simulink model "buck_mppt"  (R2020a)
settings: Solver=FixedStepAuto  StartTime=0.0  StopTime=sim_duration  FixedStep=sample_time  RelTol=1e-3
values from neighbouring files (symbols this model uses):
  Cin = 300e-6    (= 0.0003)    [main.m]
  Cout = delta_IL / (8 * fsw * delta_Vout)    (= 0.000115)    [main.m]
  delay = 0e-6    (= 0)    [main.m]
  duty_init = 0.4    [main.m]
  fsw = 1e4    (= 10000)    [main.m]
  Irradiance = 1000    [main.m]
  L = Vout * (Vin - Vout) / (delta_IL * fsw * Vin)    (= 0.000839920948617)    [main.m]
  r_small = 1e-3    (= 0.001)    [main.m]
  sample_time = 1e-6    (= 1e-06)    [main.m]
  Temperature = 25    [main.m]
  Voc = 21.9    [main.m]
  Vout = 4    [main.m]
libraries: powerlib x10, powerlib_meascontrol x3, simulink x2, re_lib x1, eePwmGenerator x1
settings Model: Creator=HP  LastModifiedBy=HP

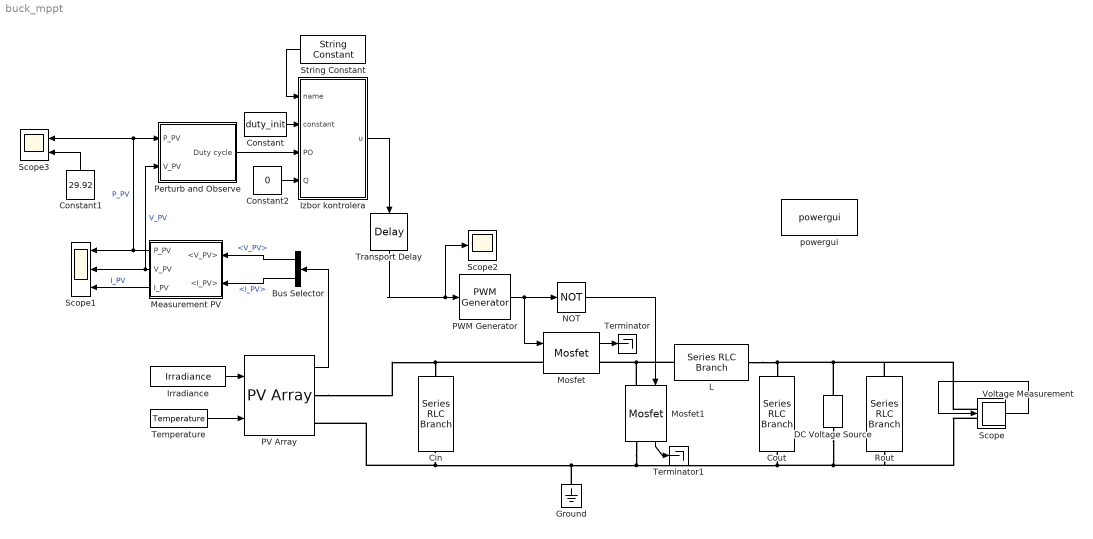
== system buck_mppt ==
  Bus Selector : BusSelector  OutputSignals=V_PV,I_PV
  Cin : powerlib/Elements/Series RLC Branch  LConnTagsString=__new0  RConnTagsString=__new0  BranchType=RC  Resistance=r_small  Inductance=L  SetiL0=off  InitialCurrent=0  Capacitance=Cin  Setx0=on  InitialVoltage=15  Measurements=None
  Constant : Constant  Value=duty_init
  Constant1 : Constant  Value=29.92
  Constant2 : Constant  Value=0
  Cout : powerlib/Elements/Series RLC Branch  LConnTagsString=__new0  RConnTagsString=__new0  BranchType=RC  Resistance=r_small  Inductance=L  SetiL0=off  InitialCurrent=0  Capacitance=Cout  Setx0=off  InitialVoltage=0  Measurements=None
  DC Voltage Source : powerlib/Electrical Sources/DC Voltage Source  Amplitude=Vout  Measurements=None
  Ground : powerlib/Elements/Ground  LConnTagsString=a
  Irradiance : Constant  Value=Irradiance
  Izbor kontrolera : Subsystem
  L : powerlib/Elements/Series RLC Branch  LConnTagsString=__new0  RConnTagsString=__new0  BranchType=RL  Resistance=r_small  Inductance=L  SetiL0=off  InitialCurrent=0  Capacitance=1e-6  Setx0=off  InitialVoltage=0  Measurements=None
  Measurement PV : Subsystem
  Mosfet : powerlib/Power Electronics/Mosfet  Ron=0.1  Lon=0  Rd=0.01  Vfd=0  IC=0  Rs=1e5  Cs=inf  Measurements=on
  Mosfet1 : powerlib/Power Electronics/Mosfet  Ron=0.1  Lon=0  Rd=0.01  Vfd=0  IC=0  Rs=1e5  Cs=inf  Measurements=on
  NOT : Logic  Operator=NOT  IconShape=distinctive  AllPortsSameDT=off  OutDataTypeStr=boolean
  PV Array : re_lib/Solar/PV Array  Npar=1  Nser=1  PlotType=array @ 1000 W/m2 & specified temperatures  S_vec="[ 1000  500  100 ]"  Temp_C_vec="[ 45 25  ]"  ModuleName=User-defined  PlotWhenSelected=off  Pm=29.92  Ncell=36  Voc=21.9  Isc=1.84  Vm=17.6  Im=1.7  beta_Voc_pc=-0.36099  alpha_Isc_pc=0.102  beta_Voc=-0.079057  alpha_Isc=0.0018768  IL=1.8445  I0=6.8285e-11  nI=0.98705  Rsh=385.9657  Rs=0.95187  RobustModel=off  RobustCellTemperature=Temperature  BAL=on  Tc=1e-6  Tfilter=5e-5
  PWM Generator : eePwmGenerator/PWM Generator  CarrCount=Up  Tper=1/fsw  Ts=sample_time
  Perturb and Observe : Subsystem
  Rout : powerlib/Elements/Series RLC Branch  LConnTagsString=__new0  RConnTagsString=__new0  BranchType=R  Resistance=1  Inductance=L  SetiL0=off  InitialCurrent=0  Capacitance=Cout  Setx0=off  InitialVoltage=0  Measurements=None
  Scope : Scope
  Scope1 : Scope  NumInputPorts=3
  Scope2 : Scope
  Scope3 : Scope  NumInputPorts=2
  String Constant : StringConstant  String=mppt_algo_name
  Temperature : Constant  Value=Temperature
  Terminator : Terminator
  Terminator1 : Terminator
  Transport Delay : TransportDelay  DelayTime=delay
  Voltage Measurement : powerlib/Measurements/Voltage Measurement  PhasorSimulation=off  OutputType=Complex  PSBequivalent=0
  powergui : powerlib/powergui  Priority=1  SimulationMode=Discrete  SampleTime=sample_time  frequency=60  Iterations=50  frequencyindice=0  Pbase=100e6  ErrMax=1e-4  UnitsV=kV  UnitsW=MW  buscounter=0  FunctionMessages=off  echomessages=off  EnableUseOfTLC=off  CurrentSourceSwitches=off  DisableSnubberDevices=off  DisableRonSwitches=off  DisableVfSwitches=off  DisplayEquations=off  AutomaticDiscreteSolvers=off  SolverType=Tustin/Backward Euler (TBE)  Interpol=off  ExternalGateDelay=off  methode=off  Ts=100  x0status=blocks  SPID=on  SwTol=0  HookPort=off  NonlinearTolerance=1e-4  nMaxIteration=100  ContinueOnMaxIteration=off  RestoreLinks=warning  ResistiveCurrentMeasurement=off  Frange=[0:2:500]  Ylog=off  Xlog=on  ShowGrid=off  save=off  variable=ZData  structure=0  ZoomFFT=off  StartTime=0.0  cycles=1  DisplayStyle=1  fundamental=60  FreqAxis=off  MaxFrequency=1000  frequencyindicesteady=1  RmsSteady=1  display=off
  wires:
  PWM Generator/1 -> NOT/1, Mosfet/1
  NOT/1 -> Mosfet1/1
  Mosfet/1 -> Terminator/1
  Mosfet1/1 -> Terminator1/1
  Voltage Measurement/1 -> Scope/1
  Irradiance/1 -> PV Array/1
  Temperature/1 -> PV Array/2
  PV Array/1 -> Bus Selector/1
  Bus Selector/1 -> Measurement PV/1(<V_PV>)  "<V_PV>"
  Bus Selector/2 -> Measurement PV/2(<I_PV>)  "<I_PV>"
  Measurement PV/1(P_PV) -> Perturb and Observe/1(P_PV), Scope3/1, Scope1/1  "P_PV"
  Measurement PV/2(V_PV) -> Perturb and Observe/2(V_PV), Scope1/2  "V_PV"
  Measurement PV/3(I_PV) -> Scope1/3  "I_PV"
  Constant1/1 -> Scope3/2
  String Constant/1 -> Izbor kontrolera/1(name)
  Constant/1 -> Izbor kontrolera/2(constant)
  Perturb and Observe/1(Duty cycle) -> Izbor kontrolera/3(PO)
  Izbor kontrolera/1(u) -> Transport Delay/1
  Transport Delay/1 -> PWM Generator/1, Scope2/1
  Constant2/1 -> Izbor kontrolera/4(Q)
  connections:
  Mosfet1/LConn1 -- L/LConn1 -- Mosfet/RConn1
  L/RConn1 -- DC Voltage Source/RConn1 -- Voltage Measurement/LConn1 -- Rout/LConn1 -- Cout/LConn1
  Cin/RConn1 -- PV Array/RConn2 -- Ground/LConn1 -- DC Voltage Source/LConn1 -- Voltage Measurement/LConn2 -- Rout/RConn1 -- Cout/RConn1 -- Mosfet1/RConn1
  Mosfet/LConn1 -- PV Array/RConn1 -- Cin/LConn1

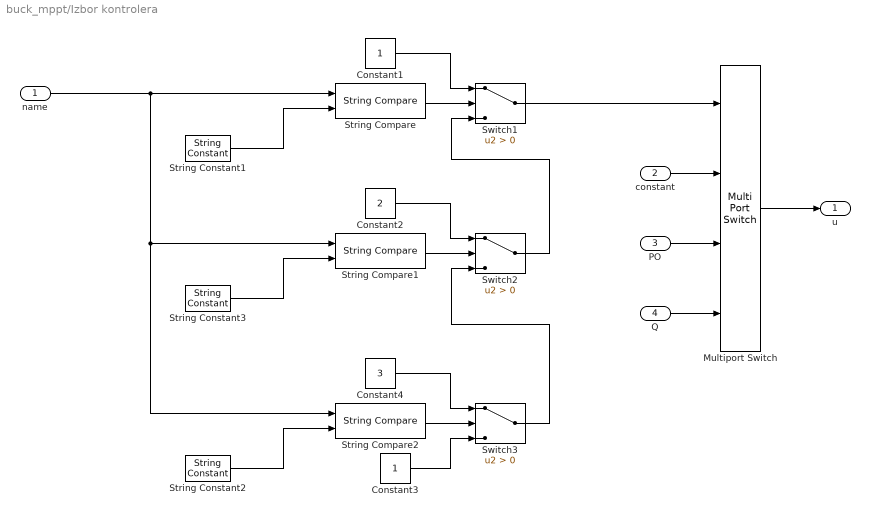
== system buck_mppt/Izbor kontrolera ==
  name : Inport
  constant : Inport  Port=2
  PO : Inport  Port=3
  Q : Inport  Port=4
  Constant1 : Constant
  Constant2 : Constant  Value=2
  Constant3 : Constant
  Constant4 : Constant  Value=3
  Multiport Switch : MultiPortSwitch
  String Compare : StringCompare
  String Compare1 : StringCompare
  String Compare2 : StringCompare
  String Constant1 : StringConstant  String="\"constant\""
  String Constant2 : StringConstant  String="\"q\""
  String Constant3 : StringConstant  String="\"po\""
  Switch1 : Switch  Criteria=u2 > Threshold
  Switch2 : Switch  Criteria=u2 > Threshold
  Switch3 : Switch  Criteria=u2 > Threshold
  u : Outport
  wires:
  String Compare1/1 -> Switch2/2
  Switch1/1 -> Multiport Switch/1
  String Constant1/1 -> String Compare/2
  String Constant3/1 -> String Compare1/2
  Constant1/1 -> Switch1/1
  Constant2/1 -> Switch2/1
  Switch2/1 -> Switch1/3
  String Compare/1 -> Switch1/2
  PO/1 -> Multiport Switch/3
  Multiport Switch/1 -> u/1
  constant/1 -> Multiport Switch/2
  Q/1 -> Multiport Switch/4
  String Compare2/1 -> Switch3/2
  String Constant2/1 -> String Compare2/2
  Constant4/1 -> Switch3/1
  Switch3/1 -> Switch2/3
  name/1 -> String Compare/1, String Compare2/1, String Compare1/1
  Constant3/1 -> Switch3/3

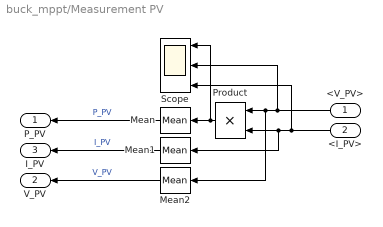
== system buck_mppt/Measurement PV ==
  <V_PV> : Inport
  <I_PV> : Inport  Port=2
  Mean : powerlib_meascontrol/Measurements/Mean  Freq=fsw  Vinit=0  Ts=0
  Mean1 : powerlib_meascontrol/Measurements/Mean  Freq=fsw  Vinit=0  Ts=0
  Mean2 : powerlib_meascontrol/Measurements/Mean  Freq=fsw  Vinit=0  Ts=0
  Product : Product
  Scope : Scope  NumInputPorts=3
  P_PV : Outport
  V_PV : Outport  Port=2
  I_PV : Outport  Port=3
  wires:
  Product/1 -> Scope/1, Mean/1
  <I_PV>/1 -> Scope/3, Mean1/1, Product/2
  <V_PV>/1 -> Scope/2, Mean2/1, Product/1
  Mean/1 -> P_PV/1  "P_PV"
  Mean1/1 -> I_PV/1  "I_PV"
  Mean2/1 -> V_PV/1  "V_PV"

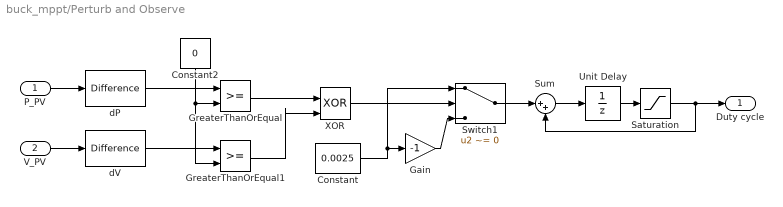
== system buck_mppt/Perturb and Observe ==
  P_PV : Inport
  V_PV : Inport  Port=2
  Constant : Constant  Value=0.0025
  Constant2 : Constant  Value=0
  Gain : Gain  Gain=-1
  GreaterThanOrEqual : RelationalOperator  OutDataTypeStr=boolean  RndMeth=Simplest
  GreaterThanOrEqual1 : RelationalOperator  OutDataTypeStr=boolean  RndMeth=Simplest
  Saturation : Saturate  UpperLimit=0.8  LowerLimit=Vout/Voc * 1.1
  Sum : Sum  Inputs=|++
  Switch1 : Switch  Criteria=u2 ~= 0
  Unit Delay : UnitDelay  InitialCondition=duty_init  SampleTime=-1  HasFrameUpgradeWarning=on
  XOR : Logic  Operator=XOR  IconShape=distinctive  AllPortsSameDT=off  OutDataTypeStr=boolean
  dP : simulink/Discrete/Difference  ICPrevInput=0.0  OutMin=[]  OutMax=[]  OutDataType=fixdt(1, 16)  OutScaling=2^-10  DoSatur=off
  dV : simulink/Discrete/Difference  ICPrevInput=0.0  OutMin=[]  OutMax=[]  OutDataType=fixdt(1, 16)  OutScaling=2^-10  DoSatur=off
  Duty cycle : Outport
  wires:
  Switch1/1 -> Sum/1
  Sum/1 -> Unit Delay/1
  Saturation/1 -> Duty cycle/1, Sum/2
  GreaterThanOrEqual1/1 -> XOR/2
  Constant/1 -> Switch1/1, Gain/1
  Constant2/1 -> GreaterThanOrEqual1/2, GreaterThanOrEqual/2
  dP/1 -> GreaterThanOrEqual/1
  XOR/1 -> Switch1/2
  dV/1 -> GreaterThanOrEqual1/1
  Unit Delay/1 -> Saturation/1
  GreaterThanOrEqual/1 -> XOR/1
  Gain/1 -> Switch1/3
  V_PV/1 -> dV/1
  P_PV/1 -> dP/1
